simulink model "Motor_MILS"  (Simulink 7.8)
settings: Solver=ode3  StartTime=0.0  StopTime=10.0  FixedStep=0.0001  MinStep=0.00001  RelTol=1e-3  AbsTol=1e-6
values from neighbouring files (symbols this model uses):
  KD = 0.45    [setup.m]
  KI = 0.7    [setup.m]
  KP = 0.8    [setup.m]
  Motor_Ke = 0.016    [setup.m]
  Motor_Kt = 0.016    [setup.m]
  Motor_L = 0.00012    [setup.m]
  Motor_R = 1.34    [setup.m]
  Rotor_Ine = 0.000000919    (= 9.19e-07)    [setup.m]
undefined symbols (not defined in the file or in its folder): sigbuilder_block
settings Model: Creator=131851  LastModifiedBy=131851
settings SolverCC: InitialStep=0.0001  MaxConsecutiveMinStep=10000
settings DataIOCC: Decimation=5  MaxDataPoints=5000

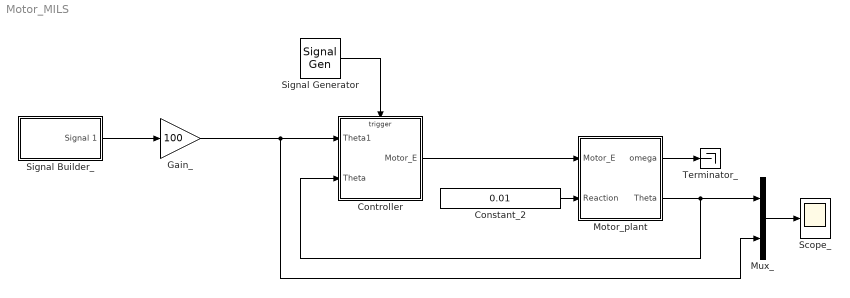
== system Motor_MILS ==
  Constant_2 : Constant  Value=0.01
      settings: AttributesFormatString=%<OutDataTypeStr>
  Controller : Subsystem
  Gain_ : Gain  Gain=100  RndMeth=Zero  SaturateOnIntegerOverflow=on
  Motor_plant : Subsystem
  Mux_ : Mux  Inputs=2
  Scope_ : Scope
      settings: SampleInput=on
  Signal Generator : SignalGenerator  WaveForm=square  Frequency=1/0.01
  Signal Builder_ : Subsystem  Tag=STV Subsys  LoadFcn=sigbuilder_block('load');  StartFcn=sigbuilder_block('start');  StopFcn=sigbuilder_block('stop');  ClipboardFcn=sigbuilder_block('clipboard');  mask(Sigbuilder block){}
      mask help: Sigbuilder GUI
      mask init:
      | if ~strcmp(get_param(bdroot(gcbh),'SimulationStatus'),'stopped') tuvar = sigbuilder_block('maskInit'); end
      settings: CopyFcn=sigbuilder_block('copy');  DeleteFcn=sigbuilder_block('delete');  ModelCloseFcn=sigbuilder_block('modelClose');  PreSaveFcn=sigbuilder_block('preSave');  NameChangeFcn=sigbuilder_block('namechange');  OpenFcn=sigbuilder_block('open',[437.25 199.5 550.5 399.75 ]);  CloseFcn=sigbuilder_block('close');
      mask Display: plot(0,0,100,100,[10,10,40,40,10],[80,20,20,80,80],[40,10],[50,50], [40,27,10],[65,72,56],[40,25,25,10],[28,28,43,43]);
  Terminator_ : Terminator
  wires:
  Signal Generator/1 -> Controller/Trigger
  Motor_plant/2(Theta) -> Controller/2(Theta), Mux_/1
  Controller/1(Motor_E) -> Motor_plant/1(Motor_E)
  Constant_2/1 -> Motor_plant/2(Reaction)
  Signal Builder_/1(Signal 1) -> Gain_/1
  Mux_/1 -> Scope_/1
  Motor_plant/1(omega) -> Terminator_/1
  Gain_/1 -> Controller/1(Theta1), Mux_/2

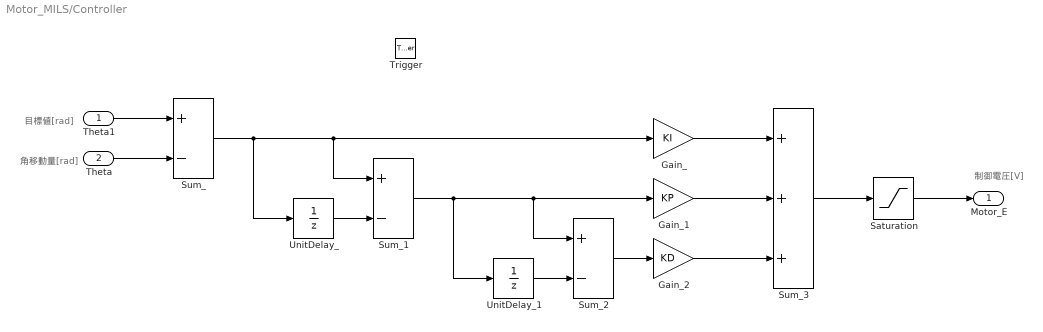
== system Motor_MILS/Controller ==
  note: 制御電圧[V]
  note: 角移動量[rad]
  note: 目標値[rad]
  Theta1 : Inport  Interpolate=off
  Theta : Inport  Port=2  Interpolate=off
  Trigger : TriggerPort  PortDimensions=1
  Gain_ : Gain  Gain=KI  RndMeth=Zero  SaturateOnIntegerOverflow=on
  Gain_1 : Gain  Gain=KP  RndMeth=Zero  SaturateOnIntegerOverflow=on
  Gain_2 : Gain  Gain=KD  RndMeth=Zero  SaturateOnIntegerOverflow=on
  Saturation : Saturate  UpperLimit=20  LowerLimit=-20
  Sum_ : Sum  Inputs=+-  RndMeth=Zero  SaturateOnIntegerOverflow=on
  Sum_1 : Sum  Inputs=+-  RndMeth=Zero  SaturateOnIntegerOverflow=on
  Sum_2 : Sum  Inputs=+-  RndMeth=Zero  SaturateOnIntegerOverflow=on
  Sum_3 : Sum  Inputs=3  RndMeth=Zero  SaturateOnIntegerOverflow=on
  UnitDelay_ : UnitDelay  SampleTime=-1
      settings: AttributesFormatString=Initial=%<x0>\nTsample=%<sampleTime>
  UnitDelay_1 : UnitDelay  SampleTime=-1
      settings: AttributesFormatString=Initial=%<x0>\nTsample=%<sampleTime>
  Motor_E : Outport
  wires:
  Theta1/1 -> Sum_/1
  Theta/1 -> Sum_/2
  Sum_/1 -> UnitDelay_/1, Gain_/1, Sum_1/1
  UnitDelay_/1 -> Sum_1/2
  Sum_1/1 -> UnitDelay_1/1, Gain_1/1, Sum_2/1
  UnitDelay_1/1 -> Sum_2/2
  Sum_2/1 -> Gain_2/1
  Gain_/1 -> Sum_3/1
  Gain_1/1 -> Sum_3/2
  Gain_2/1 -> Sum_3/3
  Saturation/1 -> Motor_E/1
  Sum_3/1 -> Saturation/1

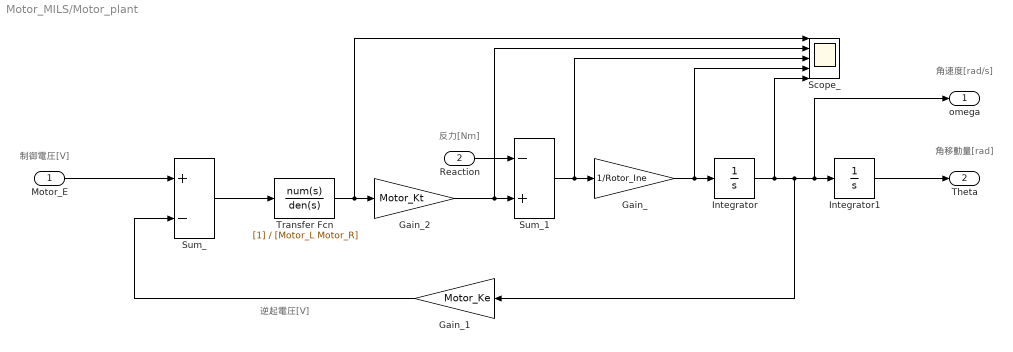
== system Motor_MILS/Motor_plant ==
  note: 制御電圧[V]
  note: 逆起電圧[V]
  note: 反力[Nm]
  note: 角移動量[rad]
  note: 角速度[rad/s]
  Motor_E : Inport  Interpolate=off
  Reaction : Inport  Port=2  Interpolate=off
  Gain_ : Gain  Gain=1/Rotor_Ine  RndMeth=Zero  SaturateOnIntegerOverflow=on
  Gain_1 : Gain  Gain=Motor_Ke  RndMeth=Zero  SaturateOnIntegerOverflow=on
  Gain_2 : Gain  Gain=Motor_Kt  OutDataTypeStr=Inherit: Inherit via back propagation  RndMeth=Zero  SaturateOnIntegerOverflow=on
  Integrator : Integrator
  Integrator1 : Integrator
  Scope_ : Scope  NumInputPorts=5
      settings: YMin=-5~-5~-5~-5~-5  YMax=5~5~5~5~5  SampleInput=on
  Sum_ : Sum  Inputs=+-  RndMeth=Zero  SaturateOnIntegerOverflow=on
  Sum_1 : Sum  Inputs=-+  RndMeth=Zero  SaturateOnIntegerOverflow=on
  Transfer Fcn : TransferFcn  Denominator=[Motor_L Motor_R]
  omega : Outport
  Theta : Outport  Port=2
  wires:
  Motor_E/1 -> Sum_/1
  Sum_/1 -> Transfer Fcn/1
  Reaction/1 -> Sum_1/1
  Sum_1/1 -> Gain_/1, Scope_/3
  Gain_/1 -> Integrator/1, Scope_/4
  Integrator/1 -> Gain_1/1, Integrator1/1, omega/1, Scope_/5
  Gain_1/1 -> Sum_/2
  Transfer Fcn/1 -> Gain_2/1, Scope_/1
  Gain_2/1 -> Sum_1/2, Scope_/2
  Integrator1/1 -> Theta/1

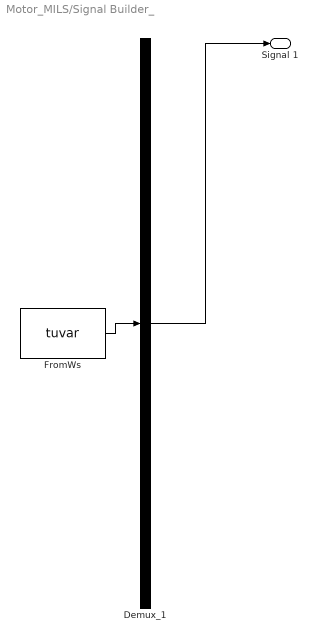
== system Motor_MILS/Signal Builder_ ==
  Demux_1 : Demux  Tag=STV Demux  Outputs=1
  FromWs : FromWorkspace  Tag=STV FromWs  VariableName=tuvar  SampleTime=0  SigBuilderData=DataTag0  VnvData=DataTag1
      SigBuilderData=|
      | common.afterFinalStr = 'Extrapolate'
      | common.sampleTime = 0
      | dataSet.timeRange = [0 10]
      | dataSet.name = 'Group 1'
      | sbobj.Groups.Name = 'Group 1'
      | sbobj.Groups.Signals.Name = 'Signal 1'
      | sbobj.Groups.Signals.XData = [0 1 1 2 2 3 3 4 5 5 5.98 6 10]
      | sbobj.Groups.Signals.YData = [0.1 0.1 0.5 0.495 0.1 0.1 0.7 1 1 0 -0.005 0.805 0]
  Signal 1 : Outport  Tag=STV Outport
  wires:
  Demux_1/1 -> Signal 1/1
  FromWs/1 -> Demux_1/1
